simulink model "predictandupdatefcn"  (R2021b)
settings: Solver=VariableStepAuto  StartTime=0  StopTime=10.0  RelTol=1e-3
model workspace (MAT data in the model file):
  T_ref = 1
libraries: slident x1, slpidlib x1
settings Model: PacingRate=1.100000  Creator=Victor  LastModifiedBy=georg
settings DataIOCC: SaveFormat=StructureWithTime
settings OptimizationCC: BlockReduction=off  BufferReuse=off  ZeroExternalMemoryAtStartup=off  ZeroInternalMemoryAtStartup=off
settings DebuggingCC: AlgebraicLoopMsg=none  UnconnectedInputMsg=none  UnconnectedOutputMsg=none  UnconnectedLineMsg=none
settings SFSimCC: SimTargetLang=C++
settings RTWCC: GenerateReport=on  LaunchReport=on  TargetLang=C++
settings GRTTargetCC: TargetLangStandard=C++11 (ISO)  CodeInterfacePackaging=C++ class

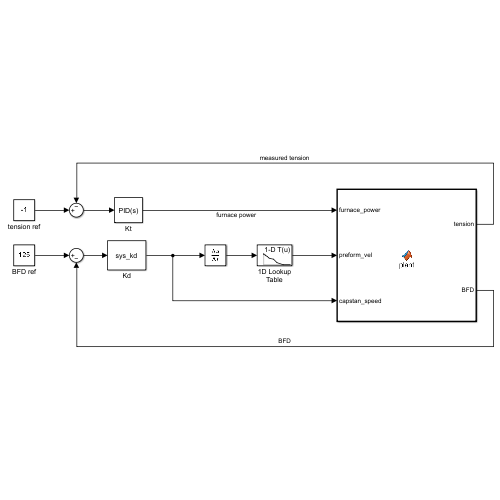
[thumbnail: Simulink's stored preview of the top-level diagram]
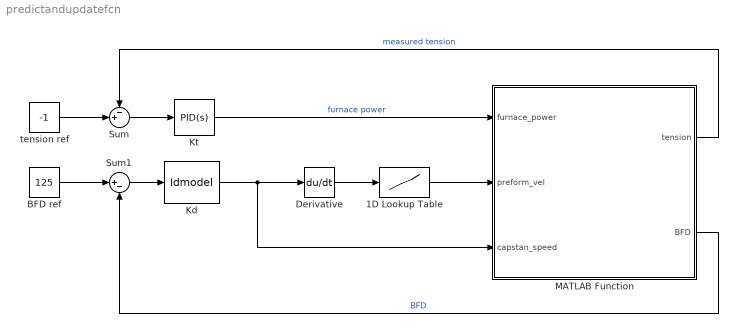
== system predictandupdatefcn ==
  1D Lookup Table : Lookup_n-D  NumberOfTableDimensions=1  BreakpointsForDimension1=[0,0.01,0.2,0.3,0.5,0.8,1,1.5,2,3,4]  Table=[2.5 2 1 0.5 -1 -2 -3 -4 -8 -10 -10]  InternalRulePriority=Speed  RndMeth=Simplest  InputSameDT=on
  BFD ref : Constant  Value=125
  Derivative : Derivative
  Kd : slident/Models/Idmodel  sys=sys_kd  IC=0  noi=on  seed=[]
      settings: SourceProductBaseCode=ID
  Kt : slpidlib/PID Controller  Controller=PID  Form=Parallel  TimeDomain=Continuous-time  UseExternalTs=off  SampleTime=-1  IntegratorMethod=Forward Euler  FilterMethod=Forward Euler  ControllerParametersSource=internal  P=0  I=0  D=1  UseFilter=on  N=100  TunerSelectOption=Transfer Function Based (PID Tuner App)  InitialConditionSource=internal  InitialConditionForIntegrator=0  InitialConditionForFilter=0  DifferentiatorICPrevScaledInput=0  ExternalReset=none  TrackingMode=off  Kt=1  LimitOutput=off  SatLimitsSource=internal  UpperSaturationLimit=inf  LowerSaturationLimit=-inf  LinearizeAsGain=on  AntiWindupMode=none  Kb=1  POutMin=[]  POutMax=[]  IOutMin=[]  IOutMax=[]  DOutMin=[]  DOutMax=[]  NOutMin=[]  NOutMax=[]  SumOutMin=[]  SumOutMax=[]  SaturationOutMin=[]  SaturationOutMax=[]  PParamMin=[]  PParamMax=[]  IParamMin=[]  IParamMax=[]  DParamMin=[]  DParamMax=[]  NParamMin=[]  NParamMax=[]  KbParamMin=[]  KbParamMax=[]  KtParamMin=[]  KtParamMax=[]  KbOutMin=[]  KbOutMax=[]  KtOutMin=[]  KtOutMax=[]  IntegratorOutMin=[]  IntegratorOutMax=[]  FilterOutMin=[]  FilterOutMax=[]  SumI1OutMin=[]  SumI1OutMax=[]  SumI2OutMin=[]  SumI2OutMax=[]  SumI3OutMin=[]  SumI3OutMax=[]  SumI4OutMin=[]  SumI4OutMax=[]  SumDOutMin=[]  SumDOutMax=[]  DifferentiatorOutMin=[]  DifferentiatorOutMax=[]  FilterDiffOutCoefMin=[]  FilterDiffOutCoefMax=[]  ReciprocalOutMin=[]  ReciprocalOutMax=[]  SumDenOutMin=[]  SumDenOutMax=[]  SumNumOutMin=[]  SumNumOutMax=[]  DivideOutMin=[]  DivideOutMax=[]  UdiffTsProdOutMin=[]  UdiffTsProdOutMax=[]  NTsProdOutMin=[]  NTsProdOutMax=[]  UintegralTsProdOutMin=[]  UintegralTsProdOutMax=[]  UngainTsProdOutMin=[]  UngainTsProdOutMax=[]  IntegratorContinuousStateAttributes=''  IntegratorStateMustResolveToSignalObject=off  IntegratorRTWStateStorageClass=Auto  FilterContinuousStateAttributes=''  FilterStateMustResolveToSignalObject=off  FilterRTWStateStorageClass=Auto  ParallelPVariant=InternalParameters  IdealPVariant=Disabled  IVariant=InternalParameters  DVariant=InternalParameters  IntegratorVariant=Continuous  SatVariant=Disabled  AWVariant=Passthrough  PCopyVariant=Disabled  TRVariant=Disabled  FdbkBlocksVariant=Forward  IdealPFdbkVariant=Disabled  SatFdbkVariant=Disabled  DerivativeFilterVariant=ContFilter  NVariant=InternalParameters  NCopyVariant=Disabled  FilterICVariant=InternalICsFilter  IntegratorICVariant=InternalICs  ExternalResetVariant=Disabled  TRSumVariant=Passthrough  SumFdbkVariant=Disabled  SumVariant=Sum_PID  TsampFilterVariant=InternalTs  TsampNgainVariant=Passthrough  TsampIntegralVariant=Passthrough  ExternalSaturationOutDataTypeStr=Inherit: Same as second input
  MATLAB Function : MATLAB Function  TreatAsAtomicUnit=on
  Sum : Sum  Inputs=-+|
  Sum1 : Sum  Inputs=|+-
  tension ref : Constant  Value=-1
  wires:
  BFD ref/1 -> Sum1/1
  MATLAB Function/2(BFD) -> Sum1/2  "BFD"
  Kd/1 -> Derivative/1, MATLAB Function/3(capstan_speed)
  Kt/1 -> MATLAB Function/1(furnace_power)  "furnace power"
  tension ref/1 -> Sum/2
  Sum/1 -> Kt/1
  MATLAB Function/1(tension) -> Sum/1  "measured tension"
  Derivative/1 -> 1D Lookup Table/1
  1D Lookup Table/1 -> MATLAB Function/2(preform_vel)
  Sum1/1 -> Kd/1

== matlab function predictandupdatefcn/MATLAB Function ==
  data: tension output; furnace_power input; preform_vel input; BFD output; capstan_speed input
function [tension, BFD] = plant(furnace_power, preform_vel, capstan_speed)
persistent model
if isempty(model)
    model = coder.loadDeepLearningNetwork("C:\Users\georg\Dropbox (MIT)\fiber-draw\run_results\architecture_experiment.mat", "deep_lstm");
end
[model, out] = model.predictAndUpdateState([furnace_power, capstan_speed, preform_vel].');
BFD = out(1);
tension = out(2);
